simulink model "lump_model_v1"  (R2024b)
settings: Solver=VariableStepAuto  StartTime=0.0  StopTime=66.5  RelTol=1e-3
model workspace (MAT data in the model file):
  A_pack = 0.4772349
  C_nominal = 3
  P = 5
  S = 138
  SoC_initial = 1
  T_amb = 301.15
  cell_Cp = 1000
  cell_mass = 0.046
  h = 5
settings Model: Creator=kara.28  LastModifiedBy=kara.28

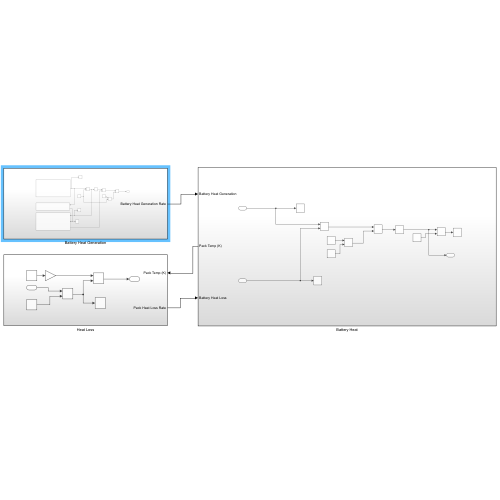
[thumbnail: Simulink's stored preview of the top-level diagram]
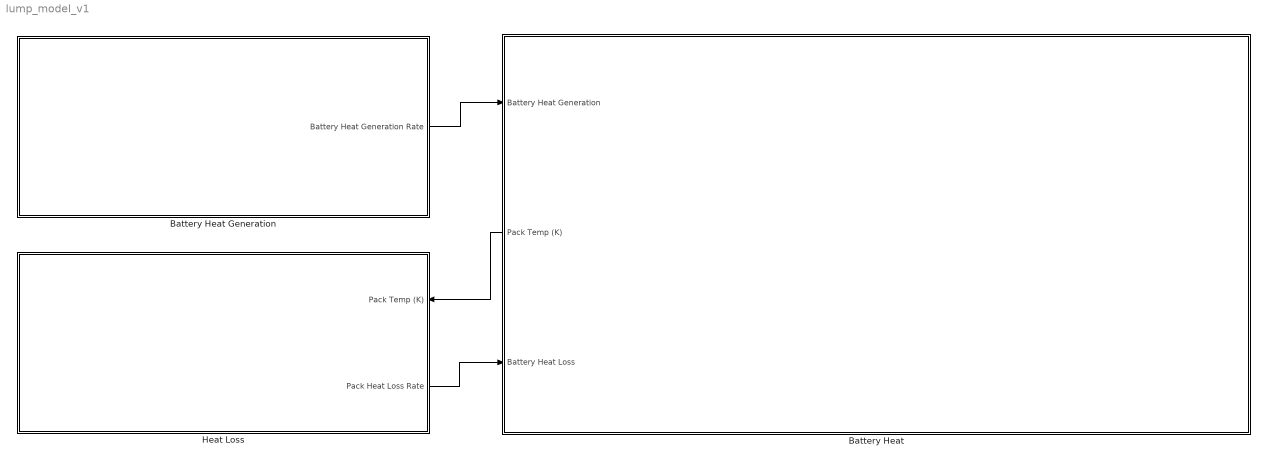
== system lump_model_v1 ==
  Battery Heat : Subsystem
      settings: PortSchema="{\"entries\":[{\"content\":{\"sides\":[{\"content\":{\"connectorIds\":[\"In1\",\"Out1\",\"In2\"]},\"type\":\"ConnectorPlacement.EquallySpacedRectSide\",\"uuid\":\"0f7c0562-63f7-413a-9c65-7d5d0f23ac53\"},{\"content\":{\"side\":\"RIGHT\"},\"type\":\"ConnectorPlacement.EquallySpacedRectSide\",\"uuid\":\"6856fc4a-e601-47fb-aafe-3183d6398fa2\"},{\"content\":{\"side\":\"TOP\"},\"type\":\"ConnectorPlacement.EquallySpacedRectSide\",\"uuid\":\"93500152-ab0c-4e86-a765-8796b82b9cd6\"}]},\"type\":\"ConnectorPlacement.EquallySpacedConnector\",\"uuid\":\"8bef09a8-0835-4033-ba4e-3f5f6277d0ac\"}],\"packageUris\":[\"http://schema.mathworks.com/mf0/Connector/R2020b\"],\"version\":\"1.0\"}"
  Battery Heat Generation : Subsystem
  Heat Loss : Subsystem
      settings: PortSchema="{\"entries\":[{\"content\":{\"sides\":[{\"content\":{},\"type\":\"ConnectorPlacement.EquallySpacedRectSide\",\"uuid\":\"cd11f8f0-ebc0-4dda-8c98-00f5919de41a\"},{\"content\":{\"connectorIds\":[\"In1\",\"Out1\"],\"side\":\"RIGHT\"},\"type\":\"ConnectorPlacement.EquallySpacedRectSide\",\"uuid\":\"2a68a9a1-bd97-4a17-8a8b-1aa98e9bd9a8\"},{\"content\":{\"side\":\"TOP\"},\"type\":\"ConnectorPlacement.EquallySpacedRectSide\",\"uuid\":\"debcc510-941b-4448-a371-f67c84c59f32\"}]},\"type\":\"ConnectorPlacement.EquallySpacedConnector\",\"uuid\":\"91559e46-754b-48b4-ac3e-ab135f9add0a\"}],\"packageUris\":[\"http://schema.mathworks.com/mf0/Connector/R2020b\"],\"version\":\"1.0\"}"
  wires:
  Battery Heat Generation/1(Battery Heat Generation Rate) -> Battery Heat/1(Battery Heat Generation)
  Heat Loss/1(Pack Heat Loss Rate) -> Battery Heat/2(Battery Heat Loss)
  Battery Heat/1(Pack Temp (K)) -> Heat Loss/1(Pack Temp (K))

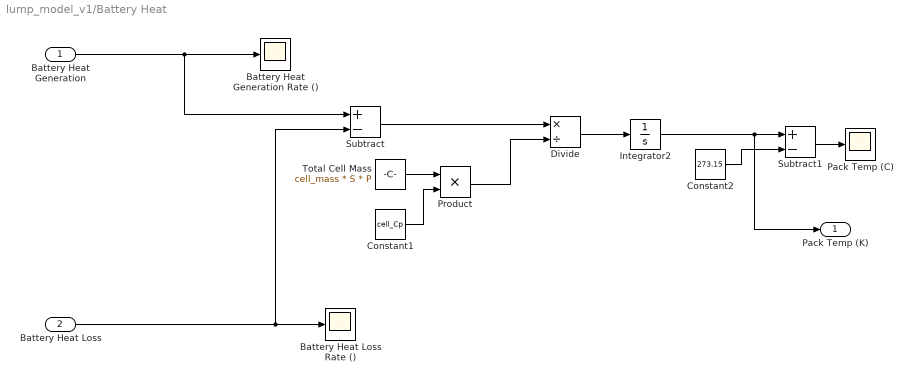
== system lump_model_v1/Battery Heat ==
  Battery Heat Generation : Inport
  Battery Heat Loss : Inport  Port=2
  Battery Heat Generation Rate () : Scope
  Battery Heat Loss Rate () : Scope
  Constant1 : Constant  Value=cell_Cp
  Constant2 : Constant  Value=273.15
  Divide : Product  Inputs=*/
  Integrator2 : Integrator  InitialCondition=T_amb
  Pack Temp (C) : Scope
  Product : Product
  Subtract : Sum  Inputs=+-
  Subtract1 : Sum  Inputs=+-
  Total Cell Mass : Constant  Value=cell_mass * S * P
  Pack Temp (K) : Outport
  wires:
  Constant1/1 -> Product/2
  Constant2/1 -> Subtract1/2
  Battery Heat Generation/1 -> Subtract/1, Battery Heat Generation Rate ()/1
  Divide/1 -> Integrator2/1
  Subtract/1 -> Divide/1
  Integrator2/1 -> Pack Temp (K)/1, Subtract1/1
  Subtract1/1 -> Pack Temp (C)/1
  Total Cell Mass/1 -> Product/1
  Product/1 -> Divide/2
  Battery Heat Loss/1 -> Battery Heat Loss Rate ()/1, Subtract/2

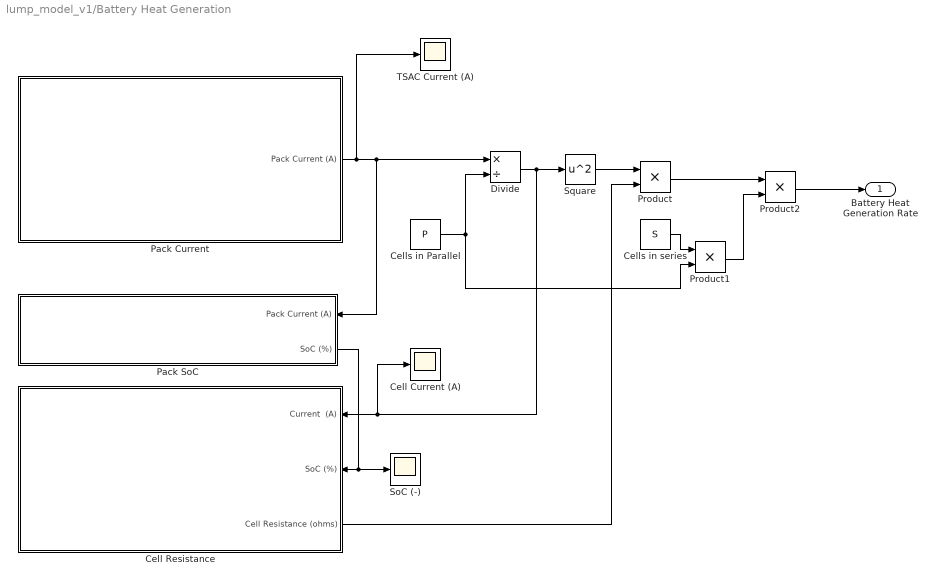
== system lump_model_v1/Battery Heat Generation ==
  Cell Current (A) : Scope
  Cell Resistance : Subsystem
      settings: PortSchema="{\"entries\":[{\"content\":{\"sides\":[{\"content\":{},\"type\":\"ConnectorPlacement.EquallySpacedRectSide\",\"uuid\":\"1c6ff2a8-2c86-4b92-aa7d-5717a02d6f28\"},{\"content\":{\"connectorIds\":[\"In1\",\"In2\",\"Out1\"],\"side\":\"RIGHT\"},\"type\":\"ConnectorPlacement.EquallySpacedRectSide\",\"uuid\":\"52a4cb2c-e1db-459d-bd0a-206cc3bba6d1\"},{\"content\":{\"side\":\"TOP\"},\"type\":\"ConnectorPlacement.EquallySpacedRectSide\",\"uuid\":\"751bbbd6-abc7-4265-8d68-4aa70d69379f\"}]},\"type\":\"ConnectorPlacement.EquallySpacedConnector\",\"uuid\":\"b8f9630f-0167-4478-8d98-637e13782dcd\"}],\"packageUris\":[\"http://schema.mathworks.com/mf0/Connector/R2020b\"],\"version\":\"1.0\"}"
  Cells in Parallel : Constant  Value=P
  Cells in series : Constant  Value=S
  Divide : Product  Inputs=*/
  Pack Current : Subsystem
  Pack SoC : Subsystem
      settings: PortSchema="{\"entries\":[{\"content\":{\"sides\":[{\"content\":{},\"type\":\"ConnectorPlacement.EquallySpacedRectSide\",\"uuid\":\"1c6ff2a8-2c86-4b92-aa7d-5717a02d6f28\"},{\"content\":{\"connectorIds\":[\"In1\",\"Out1\"],\"side\":\"RIGHT\"},\"type\":\"ConnectorPlacement.EquallySpacedRectSide\",\"uuid\":\"52a4cb2c-e1db-459d-bd0a-206cc3bba6d1\"},{\"content\":{\"side\":\"TOP\"},\"type\":\"ConnectorPlacement.EquallySpacedRectSide\",\"uuid\":\"751bbbd6-abc7-4265-8d68-4aa70d69379f\"}]},\"type\":\"ConnectorPlacement.EquallySpacedConnector\",\"uuid\":\"b8f9630f-0167-4478-8d98-637e13782dcd\"}],\"packageUris\":[\"http://schema.mathworks.com/mf0/Connector/R2020b\"],\"version\":\"1.0\"}"
  Product : Product
  Product1 : Product
  Product2 : Product
  SoC (-) : Scope
  Square : Math  Operator=square
  TSAC Current (A) : Scope
  Battery Heat Generation Rate : Outport
  wires:
  Pack Current/1(Pack Current (A)) -> TSAC Current (A)/1, Pack SoC/1(Pack Current (A)), Divide/1
  Cells in series/1 -> Product1/1
  Divide/1 -> Cell Current (A)/1, Cell Resistance/1(Current  (A)), Square/1
  Cell Resistance/1(Cell Resistance (ohms)) -> Product/2
  Square/1 -> Product/1
  Cells in Parallel/1 -> Divide/2, Product1/2
  Product1/1 -> Product2/2
  Product/1 -> Product2/1
  Product2/1 -> Battery Heat Generation Rate/1
  Pack SoC/1(SoC (%)) -> SoC (-)/1, Cell Resistance/2(SoC (%))

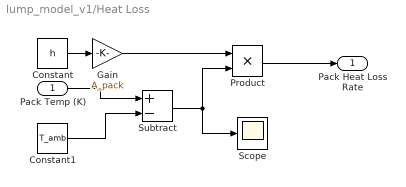
== system lump_model_v1/Heat Loss ==
  Pack Temp (K) : Inport
  Constant : Constant  Value=h
  Constant1 : Constant  Value=T_amb
  Gain : Gain  Gain=A_pack
  Product : Product
  Scope : Scope
  Subtract : Sum  Inputs=+-
  Pack Heat Loss Rate : Outport
  wires:
  Constant/1 -> Gain/1
  Subtract/1 -> Product/2, Scope/1
  Gain/1 -> Product/1
  Product/1 -> Pack Heat Loss Rate/1
  Pack Temp (K)/1 -> Subtract/1
  Constant1/1 -> Subtract/2

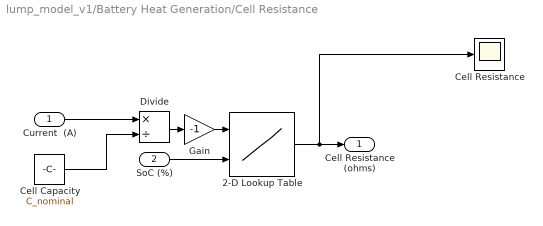
== system lump_model_v1/Battery Heat Generation/Cell Resistance ==
  Current  (A) : Inport
  SoC (%) : Inport  Port=2
  2-D Lookup Table : Lookup_n-D  BreakpointsForDimension1=[-10;-5;-1;1;2;3]  BreakpointsForDimension2=[0.1;0.2;0.3;0.4;0.5;0.6;0.7;0.8;0.9;1]  Table=[0.018906 0.01868 0.018453 0.018226 0.017999 0.017916 0.017743 0.018183 0.019549 0.022703;0.021356 0.020344 0.019332 0.019017 0.018694 0.018598 0.018319 0.018773 0.020642 0.024917;0.02305 0.020909 0.018859 0.019644 0.019687 0.018989 0.018291 0.019295 0.021608 0.026536;0.023001 0.020599 0.019683 0.019161 0.01894 0.018506 0.018636 0.019336 0.020993 0.02265;0.022654 0.020712 0.018901 0.018682 0.018442 0.018289 0.017788 0.017286 0.016785 0.016283;0.019898 0.017891 0.017366 0.01725 0.01725 0.017251 0.017251 0.017251 0.017251 0.017251]  InterpMethod=Cubic spline  ExtrapMethod=Clip  InternalRulePriority=Speed  RndMeth=Simplest
      settings: InputPortMap=u0,u1
  Cell Capacity : Constant  Value=C_nominal
  "Cell Resistance " : Scope
  Divide : Product  Inputs=*/
  Gain : Gain  Gain=-1
  Cell Resistance (ohms) : Outport
  wires:
  Current  (A)/1 -> Divide/1
  Cell Capacity/1 -> Divide/2
  SoC (%)/1 -> 2-D Lookup Table/2
  2-D Lookup Table/1 -> "Cell Resistance "/1, Cell Resistance (ohms)/1
  Divide/1 -> Gain/1
  Gain/1 -> 2-D Lookup Table/1

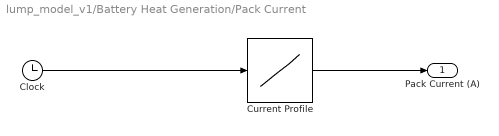
== system lump_model_v1/Battery Heat Generation/Pack Current ==
  Clock : Clock
  Current Profile : Lookup_n-D  NumberOfTableDimensions=1  BreakpointsForDimension1=[0;0.97380699999999998;1.456439;1.923767;2.3677250000000001;2.7497120000000002;3.0680339999999999;3.342889;3.5899269999999999;3.8181120000000002;4.030875;4.2442669999999998;4.4751950000000003;4.7151730000000001;4.954453;5.1887489999999996;5.4100169999999999;5.6180009999999996;5.8186020000000003;6.0121289999999998;6.1999810000000002;6.3869670000000003;6.5739520000000002;6.7609380000000003;6.9479240000000004;7.1349090000000004;7.3218949999999996;7.5088800000000004;7.6958659999999997;7.8828509999999996;8.0698369999999997;8.2568230000000007;8.4438089999999999;8.6307939999999999;8.8177800000000008;9.0047650000000008;9.191751;9.378736;9.5657219999999992;9.7527069999999991;9.9396920000000009;10.12668;10.31366;10.50065;10.68764;10.87462;11.06161;11.24859;11.43558;11.62256;11.80955;11.99653;12.18352;12.370509999999999;12.55749;12.744479999999999;12.93146;13.118449999999999;13.305429999999999;13.492419999999999;13.679399999999999;13.866390000000001;14.053380000000001;14.240360000000001;14.427350000000001;14.614330000000001;14.80132;14.988300000000001;15.17529;15.362270000000001;15.54926;15.73625;15.92323;16.110220000000002;16.2972;16.484190000000002;16.67117;16.858160000000002;17.049309999999998;17.256350000000001;17.490680000000001;17.72842;17.954529999999998;18.18882;18.430389999999999;18.670480000000001;18.9055;19.127289999999999;19.340949999999999;19.5519;19.75929;19.965440000000001;20.16865;20.36543;20.557880000000001;20.747129999999999;20.93412;21.121099999999998;21.30809;21.495080000000002;21.68206;21.869050000000001;22.05603;22.243020000000001;22.43;22.616990000000001;22.80397;22.990960000000001;23.177949999999999;23.364930000000001;23.551919999999999;23.738900000000001;23.925889999999999;24.119759999999999;24.33417;24.58145;24.870660000000001;25.1874;25.501380000000001;25.809709999999999;26.106909999999999;26.396740000000001;26.672989999999999;26.934360000000002;27.195170000000001;27.44707;27.68083;27.91536;28.178429999999999;28.484400000000001;28.839289999999998;29.22064;29.59496;29.961099999999998;30.31212;30.641480000000001;30.953890000000001;31.274570000000001;31.640139999999999;32.029879999999999;32.414169999999999;32.79468;33.141350000000003;33.432960000000001;33.685090000000002;33.923769999999998;34.157600000000002;34.378779999999999;34.588009999999997;34.787269999999999;34.991610000000001;35.215609999999998;35.447719999999997;35.679299999999998;35.906440000000003;36.121899999999997;36.332729999999998;36.560650000000003;36.824579999999997;37.131489999999999;37.456029999999998;37.774590000000003;38.079030000000003;38.36007;38.621299999999998;38.869950000000003;39.113210000000002;39.354239999999997;39.589770000000001;39.811239999999998;40.018039999999999;40.218699999999998;40.418289999999999;40.615740000000002;40.80735;40.99436;41.181339999999999;41.36833;41.555309999999999;41.7423;41.929290000000002;42.11627;42.303260000000002;42.49024;42.677230000000002;42.86421;43.051200000000001;43.238190000000003;43.425170000000001;43.612160000000003;43.799140000000001;43.986130000000003;44.173110000000001;44.360619999999997;44.554279999999999;44.766030000000001;45.006309999999999;45.249270000000003;45.47945;45.724240000000002;45.970440000000004;46.215820000000001;46.494210000000002;46.791690000000003;47.086570000000002;47.36448;47.62144;47.872810000000001;48.11795;48.347279999999998;48.565379999999998;48.791339999999998;49.044379999999997;49.322989999999997;49.604320000000001;49.88111;50.148620000000001;50.404559999999996;50.668019999999999;50.94744;51.236840000000001;51.532389999999999;51.825780000000002;52.116160000000001;52.3947;52.654539999999997;52.915550000000003;53.181220000000003;53.442599999999999;53.702089999999998;53.950659999999999;54.179989999999997;54.3919;54.59104;54.781860000000002;54.972729999999999;55.177460000000004;55.410119999999999;55.677379999999999;55.96161;56.244100000000003;56.535139999999998;56.809640000000002;57.065750000000001;57.348050000000001;57.656840000000003;57.964759999999998;58.264049999999997 ...(+474 chars)]  Table=[0;5.5025339999999998;144.25659999999999;144.74039999999999;144.77070000000001;144.7748;144.77719999999999;144.77940000000001;144.78129999999999;144.78309999999999;144.78479999999999;0;0;0;144.25059999999999;144.75700000000001;144.78800000000001;144.79140000000001;144.79320000000001;144.79480000000001;144.7963;144.7979;144.79949999999999;144.80099999999999;144.80260000000001;144.80410000000001;144.8056;144.80719999999999;144.80879999999999;144.81030000000001;144.81190000000001;144.8134;144.815;144.81649999999999;144.81809999999999;144.81960000000001;144.8212;144.8227;144.82429999999999;144.82579999999999;144.82740000000001;144.8289;144.8305;144.83199999999999;144.83359999999999;144.83510000000001;144.83670000000001;144.8382;144.8398;144.84129999999999;144.84289999999999;144.84450000000001;144.846;144.8475;144.84909999999999;144.85069999999999;144.85220000000001;144.85380000000001;144.8553;144.8569;144.85839999999999;144.86000000000001;144.86150000000001;144.8631;144.8646;144.86619999999999;144.86770000000001;144.86930000000001;144.8708;144.8724;144.87389999999999;144.87549999999999;144.87710000000001;144.87860000000001;144.8802;144.8817;144.88329999999999;144.88480000000001;0;0;0;0;144.34880000000001;0;0;144.35059999999999;144.8587;144.88980000000001;144.89330000000001;144.89510000000001;144.89670000000001;144.89850000000001;144.90010000000001;144.90180000000001;144.9034;144.905;144.9066;144.90809999999999;144.90969999999999;144.91120000000001;144.9128;144.9143;144.91589999999999;144.91739999999999;144.91900000000001;144.92060000000001;144.9221;144.9237;144.92519999999999;144.92679999999999;144.92830000000001;144.9299;144.9314;0;0;0;0;0;144.3946;144.9034;144.93520000000001;144.93940000000001;144.9418;144.94399999999999;144.94630000000001;144.9485;144.95070000000001;0;0;0;0;0;144.4143;144.92339999999999;144.95580000000001;144.96039999999999;144.9632;0;0;0;144.42769999999999;144.93700000000001;144.9691;144.9735;144.976;144.97810000000001;144.97989999999999;144.98169999999999;144.98339999999999;144.98509999999999;0;0;0;144.44739999999999;144.95699999999999;144.98820000000001;144.99160000000001;0;0;0;0;144.45400000000001;144.96379999999999;144.99539999999999;144.99930000000001;145.00139999999999;145.0034;145.00540000000001;145.00739999999999;145.0093;145.0112;145.0129;145.0146;145.01609999999999;144.57640000000001;144.99369999999999;145.01929999999999;145.0223;145.0239;145.02549999999999;145.02709999999999;145.02860000000001;145.03020000000001;145.0317;145.0333;145.03489999999999;145.03639999999999;145.03800000000001;145.0395;145.0411;145.04259999999999;145.04419999999999;145.04570000000001;0;0;0;0;0;144.5069;0;0;144.50880000000001;0;0;144.51079999999999;145.0214;145.0531;145.05690000000001;145.0591;145.06110000000001;145.06290000000001;0;0;0;0;144.5241;145.035;145.0667;0;0;0;0;144.5301;145.0411;145.07300000000001;145.0771;0;0;144.53899999999999;145.05009999999999;145.08179999999999;145.0857;145.08779999999999;145.08969999999999;145.09139999999999;0;0;0;0;0;144.55179999999999;0;144.5538;145.0652;0;0;144.5582;145.06960000000001;145.10130000000001;0;144.565;145.07650000000001;145.10830000000001;0;0;144.57140000000001;145.083;0;0;144.5762;145.08799999999999;0;0;144.58150000000001;0;0;144.584;145.0959;145.12860000000001;145.13329999999999;145.1362;145.13849999999999;0;0]  DiagnosticForOutOfRangeInput=Error  InternalRulePriority=Speed  RndMeth=Simplest
  Pack Current (A) : Outport
  wires:
  Clock/1 -> Current Profile/1
  Current Profile/1 -> Pack Current (A)/1

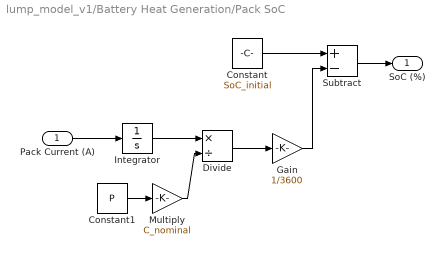
== system lump_model_v1/Battery Heat Generation/Pack SoC ==
  Pack Current (A) : Inport
  Constant : Constant  Value=SoC_initial
  Constant1 : Constant  Value=P
  Divide : Product  Inputs=*/
  Gain : Gain  Gain=1/3600
  Integrator : Integrator
  Multiply : Gain  Gain=C_nominal
  Subtract : Sum  Inputs=+-
  SoC (%) : Outport
  wires:
  Pack Current (A)/1 -> Integrator/1
  Constant/1 -> Subtract/1
  Integrator/1 -> Divide/1
  Subtract/1 -> SoC (%)/1
  Constant1/1 -> Multiply/1
  Multiply/1 -> Divide/2
  Divide/1 -> Gain/1
  Gain/1 -> Subtract/2
